simulink model "Pendulum_ViscousDamping"  (R2024a)
settings: Solver=VariableStepAuto  StartTime=0.0  StopTime=10  MaxStep=0.01  RelTol=1e-3
settings Model: Creator=Shubhada
settings SolverCC: AlgebraicLoopSolver=TrustRegion
settings DataIOCC: ExternalInput=data  LoadExternalInput=on  SaveFormat=Array  DSMLogging=off  ReturnWorkspaceOutputs=off
settings DebuggingCC: UnconnectedInputMsg=warning  UnconnectedOutputMsg=warning  UnconnectedLineMsg=warning
settings ModelReferenceCC: EnableRefExpFcnMdlSchedulingChecks=on
settings SFSimCC: CustomCodeUndefinedFunction=UseInterfaceOnly
settings RTWCC: GPUComputeCapability=3.5

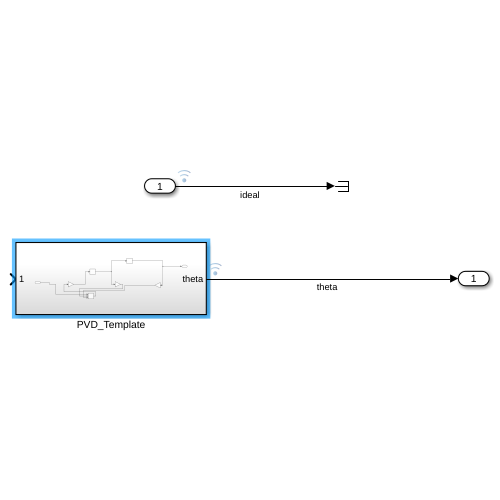
[thumbnail: Simulink's stored preview of the top-level diagram]
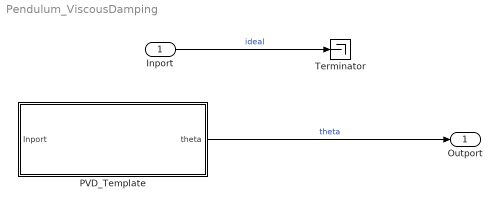
== system Pendulum_ViscousDamping ==
  Inport : Inport
  PVD_Template : Subsystem
  Terminator : Terminator
  Outport : Outport
  wires:
  PVD_Template/1(theta) -> Outport/1  "theta"
  Inport/1 -> Terminator/1  "ideal"

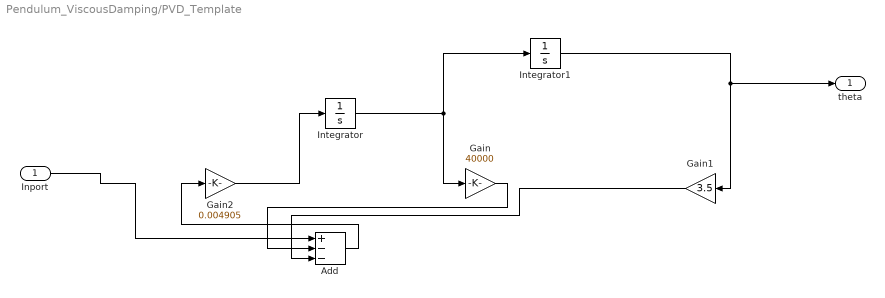
== system Pendulum_ViscousDamping/PVD_Template ==
  Inport : Inport
  Add : Sum  Inputs=+--
  Gain : Gain  Gain=40000
  Gain1 : Gain  Gain=3.5
  Gain2 : Gain  Gain=0.004905
  Integrator : Integrator
  Integrator1 : Integrator
  theta : Outport
  wires:
  Gain2/1 -> Integrator/1
  Gain1/1 -> Add/3
  Gain/1 -> Add/2
  Integrator/1 -> Gain/1, Integrator1/1
  Integrator1/1 -> Gain1/1, theta/1
  Inport/1 -> Add/1
  Add/1 -> Gain2/1
